simulink model "M2_chart_3_function_call"  (R2024a)
settings: Solver=FixedStepDiscrete  StartTime=0.0  StopTime=10.0  FixedStep=0.001  RelTol=1e-3  EnableMultiTasking=on
libraries: simulink x1
settings Model: Creator=saura  LastModifiedBy=Ishant
settings SolverCC: AlgebraicLoopSolver=TrustRegion  AutoInsertRateTranBlk=on
settings DataIOCC: LimitDataPoints=on
settings OptimizationCC: LifeSpan=inf
settings DebuggingCC: UnconnectedInputMsg=warning  UnconnectedOutputMsg=warning  UnconnectedLineMsg=warning  AllowSymbolicDim=off  SFUnexpectedBacktrackingDiag=warning  SFNoUnconditionalDefaultTransitionDiag=warning  SFExecutionAtInitializationDiag=none  ArithmeticOperatorsInVariantConditions=warning
settings ModelReferenceCC: EnableRefExpFcnMdlSchedulingChecks=on
settings SFSimCC: SimUseLocalCustomCode=off  CustomCodeUndefinedFunction=UseInterfaceOnly
settings RTWCC: RTWUseLocalCustomCode=off  GPUComputeCapability=3.5  DLArmComputeVersion=19.05
settings CodeAppCC: StateflowObjectComments=on
settings GRTTargetCC: TargetLangStandard=C89/C90 (ANSI)
settings ConfigComp: CovMetricSettings=dw  CovSaveCumulativeToWorkspaceVar=on  CovSaveSingleToWorkspaceVar=on  CovExternalEMLEnable=off  CovSFcnEnable=off

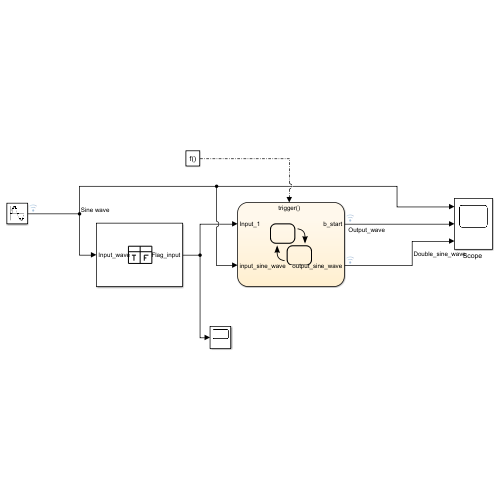
[thumbnail: Simulink's stored preview of the top-level diagram]
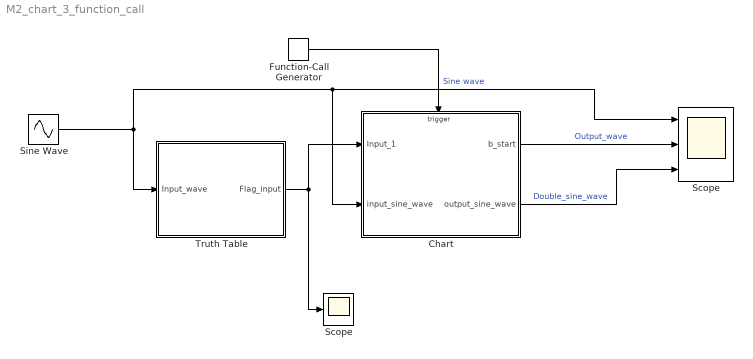
== system M2_chart_3_function_call ==
  Chart : Stateflow chart  TreatAsAtomicUnit=on
  Function-Call Generator : simulink/Ports & Subsystems/Function-Call Generator  sample_time=0.001  numberOfIterations=1  DisallowWideOutput=off
  Scope : Scope
  "Scope " : Scope  NumInputPorts=3
  Sine Wave : Sin
  Truth Table : Truth Table  TreatAsAtomicUnit=on
  wires:
  Sine Wave/1 -> "Scope "/1, Chart/2(input_sine_wave), Truth Table/1(Input_wave)  "Sine wave"
  Truth Table/1(Flag_input) -> Scope/1, Chart/1(Input_1)
  Chart/1(b_start) -> "Scope "/2  "Output_wave"
  Chart/2(output_sine_wave) -> "Scope "/3  "Double_sine_wave"
  Function-Call Generator/1 -> Chart/Trigger

== matlab function M2_chart_3_function_call/Truth Table ==
  data: Input_wave input; Flag_input output
function Flag_input = fcn(Input_wave)

aVarTruthTableCondition_1 = false;
aVarTruthTableCondition_2 = false;


% condition2

aVarTruthTableCondition_1 = logical(Input_wave<=0.5);

% condition 1

aVarTruthTableCondition_2 = logical(Input_wave >0.5);

if (aVarTruthTableCondition_2)
    aFcnTruthTableAction_2();
elseif (aVarTruthTableCondition_1)
    aFcnTruthTableAction_1();
else % Default
    aFcnTruthTableAction_3();
end

function aFcnTruthTableAction_1()

% Example action 1 called from D2 column in condition table

Flag_input = 1;

function aFcnTruthTableAction_2()

% Example action 2 called from D1 column in condition table

Flag_input = -1

function aFcnTruthTableAction_3()

% nothing

Flag_input =0

== stateflow chart M2_chart_3_function_call/Chart ==
  state master
    state base [parallel]
      en:
      b_start=-1;
      settings: executionOrder=1
      state On
        en:
        during:
        b_start=1;
      state Off
        during:
        b_start=-1;
      (default) -> On
      On -> Off : [Input_1==1]
      Off -> On : [Input_1==-1]
    state double [parallel]
      during:
      output_sine_wave=2*input_sine_wave;
      settings: executionOrder=2
  data: data local; b_start output double; Input_1 input double; input_sine_wave input double; output_sine_wave output double
  events: trigger input FUNCTION_CALL_EVENT
